simulink model "Sqrt"  (R2020a)
settings: Solver=VariableStepAuto  StartTime=0.0  StopTime=10.0  RelTol=1e-3
settings Model: Creator=royde  LastModifiedBy=royde

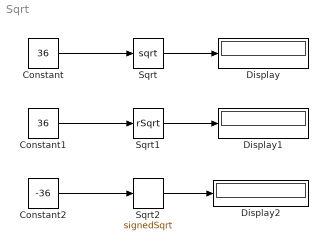
== system Sqrt ==
  Constant : Constant  Value=36
  Constant1 : Constant  Value=36
  Constant2 : Constant  Value=-36
  Display : Display
  Display1 : Display
  Display2 : Display
  Sqrt : Sqrt  SaturateOnIntegerOverflow=on
  Sqrt1 : Sqrt  Operator=rSqrt  SaturateOnIntegerOverflow=on
  Sqrt2 : Sqrt  Operator=signedSqrt  OutputSignalType=complex  SaturateOnIntegerOverflow=on
  wires:
  Constant/1 -> Sqrt/1
  Constant1/1 -> Sqrt1/1
  Constant2/1 -> Sqrt2/1
  Sqrt/1 -> Display/1
  Sqrt1/1 -> Display1/1
  Sqrt2/1 -> Display2/1
